simulink model "question5"  (R2024b)
settings: Solver=VariableStepAuto  StartTime=0.0  StopTime=10  RelTol=1e-3
model workspace (MAT data in the model file):
  C = 1
  L = 1
  R = 0.25
settings Model: Creator=marti  LastModifiedBy=marti

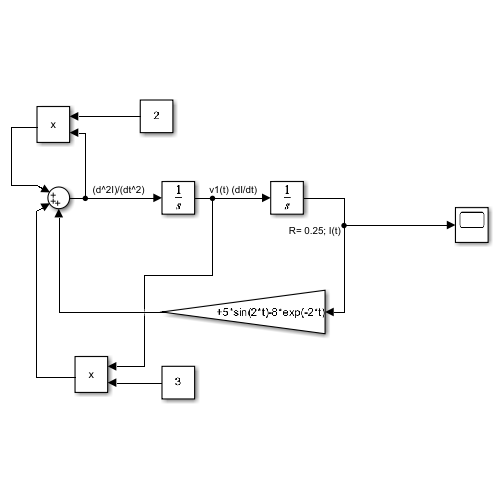
[thumbnail: Simulink's stored preview of the top-level diagram]
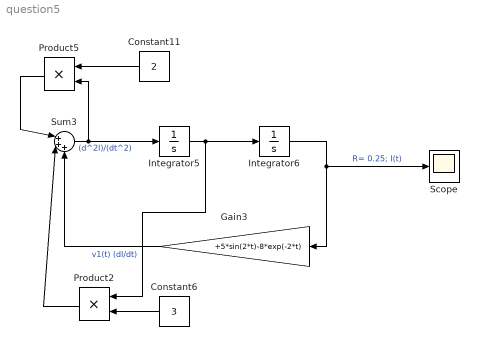
== system question5 ==
  Constant11 : Constant  Value=2
  Constant6 : Constant  Value=3
  Gain3 : Gain  Gain=+5*sin(2*t)-8*exp(-2*t)
  Integrator5 : Integrator
  Integrator6 : Integrator  InitialCondition=2
  Product2 : Product
  Product5 : Product
  Scope : Scope
  Sum3 : Sum  Inputs=|+++
  wires:
  Integrator5/1 -> Product2/1, Integrator6/1  "v1(t) (dI/dt)"
  Integrator6/1 -> Scope/1, Gain3/1  "R= 0.25; I(t)"
  Sum3/1 -> Product5/2, Integrator5/1  "(d^2I)/(dt^2)"
  Product2/1 -> Sum3/2
  Constant6/1 -> Product2/2
  Gain3/1 -> Sum3/3
  Constant11/1 -> Product5/1
  Product5/1 -> Sum3/1
